simulink model "mrefrobotarm_previous_y_previous_u_previous_ref_cex_2"  (R2018b)
settings: Solver=FixedStepAuto  StartTime=0.0  StopTime=20  RelTol=1e-3  AbsTol=1e-6
undefined symbols (not defined in the file or in its folder): cc, options
libraries: neural x462, simulink x2
(part 14 of 18)

== system mrefrobotarm_previous_y_previous_u_previous_ref_cex_2/no_cex/Layer 3/Delays 1 ==
  "p{3}" : Inport  PortDimensions=30
      mask Display: e = 0.06;c1 = [120 230 180]/255;c2 = ([120 230 180]+0)/(256+128);c3 = ([120 230 180]+128)/(256+128);patch([0 1 1 0],[0 0 1 1],c1);patch([0 1 1 1-e 1-e 0+e],[0 0 1 1-e 0+e 0+e],c2);patch([0 0 1 1-e 0+e 0+e],[0 1 1 1-e 1-e 0+e],c3);plot([0 1 1 0 0],[0 0 1 1 0]);
  mux : Mux  Inputs=1
      mask Display: e = 0.06;c1 = [120 150 230]/255;c2 = ([120 150 230]+0)/383;c3 = ([120 150 230]+128)/383;patch([0 1 1 0],[0 0 1 1],c1);patch([0 1 1 1-e 1-e 0+e],[0 0 1 1-e 0+e 0+e],c2);patch([0 0 1 1-e 0+e 0+e],[0 1 1 1-e 1-e 0+e],c3);plot([0 1 1 0 0],[0 0 1 1 0]);disp('Mux')
  "pd{3,2}" : Outport
      mask Display: e = 0.06;c1 = [120 230 180]/255;c2 = ([120 230 180]+0)/(256+128);c3 = ([120 230 180]+128)/(256+128);patch([0 1 1 0],[0 0 1 1],c1);patch([0 1 1 1-e 1-e 0+e],[0 0 1 1-e 0+e 0+e],c2);patch([0 0 1 1-e 0+e 0+e],[0 1 1 1-e 1-e 0+e],c3);plot([0 1 1 0 0],[0 0 1 1 0]);
  wires:
  "p{3}"/1 -> mux/1
  mux/1 -> "pd{3,2}"/1

== system mrefrobotarm_previous_y_previous_u_previous_ref_cex_2/no_cex/Layer 3/LW{3,2} ==
  "ad{3,2}" : Inport  PortDimensions=30
      mask Display: e = 0.06;c1 = [120 230 180]/255;c2 = ([120 230 180]+0)/(256+128);c3 = ([120 230 180]+128)/(256+128);patch([0 1 1 0],[0 0 1 1],c1);patch([0 1 1 1-e 1-e 0+e],[0 0 1 1-e 0+e 0+e],c2);patch([0 0 1 1-e 0+e 0+e],[0 1 1 1-e 1-e 0+e],c3);plot([0 1 1 0 0],[0 0 1 1 0]);
  "IW{3,2}(1,:)'" : Constant  Value=[-0.179633159964680266806880126750911585986614227294921875;-0.01072873765062364037614628387018456123769283294677734375;-0.0291453057248748058360998669513719505630433559417724609375;0.05859045612955075810202032471352140419185161590576171875;-0.237638764700321913903025006220559589564800262451171875;-0.209838527725091539277713081901310943067073822021484375;-0.27791655307496510030063063823035918176174163818359375;-0.07008976059233355815347721318175899796187877655029296875;-0.11554327471293225626514100667918683029711246490478515625;0.27212249906517038677833397741778753697872161865234375;-0.1734031338030869451305449047140427865087985992431640625;0.0536763624525791460673218580268439836800098419189453125;-0.037173437880853761605681739865758572705090045928955078125;0.1358518131119930971717479906146763823926448822021484375;-0.11157815841815578450368917629020870663225650787353515625;-0.023913464068717076027592582931902143172919750213623046875;-0.4313994517536372530486232790281064808368682861328125;0.1636875861604869808463291747102630324661731719970703125;0.037232113811342650022684352961732656694948673248291015625;-0.52644415726454052428806562602403573691844940185546875;0.039897217969779720514456045066253864206373691558837890625;-0.1369287872106144388073545314910006709396839141845703125;0.44593864887069745162051503939437679946422576904296875;0.410742338437982856813590615274733863770961761474609375;-0.145121658875231818175421949490555562078952789306640625;0.06655502995710448066457587401600903831422328948974609375;-0.418109406113754300537976860141498036682605743408203125;0.11096998879556761730125202802810235880315303802490234375;0.333827163986122277261614499366260133683681488037109375;0.186101897373585012385177606120123527944087982177734375]
      mask Display: e = 0.06;c1 = [120 150 230]/255;c2 = ([120 150 230]+0)/383;c3 = ([120 150 230]+128)/383;patch([0 1 1 0],[0 0 1 1],c1);patch([0 1 1 1-e 1-e 0+e],[0 0 1 1-e 0+e 0+e],c2);patch([0 0 1 1-e 0+e 0+e],[0 1 1 1-e 1-e 0+e],c3);plot([0 1 1 0 0],[0 0 1 1 0]);disp('weights');
  Mux : Mux  Inputs=1
      mask Display: e = 0.06;c1 = [120 150 230]/255;c2 = ([120 150 230]+0)/383;c3 = ([120 150 230]+128)/383;patch([0 1 1 0],[0 0 1 1],c1);patch([0 1 1 1-e 1-e 0+e],[0 0 1 1-e 0+e 0+e],c2);patch([0 0 1 1-e 0+e 0+e],[0 1 1 1-e 1-e 0+e],c3);plot([0 1 1 0 0],[0 0 1 1 0]);disp('Mux');
  dotprod1 : neural/Weight Functions/dotprod
  "lz{3,2}" : Outport
      mask Display: e = 0.06;c1 = [120 230 180]/255;c2 = ([120 230 180]+0)/(256+128);c3 = ([120 230 180]+128)/(256+128);patch([0 1 1 0],[0 0 1 1],c1);patch([0 1 1 1-e 1-e 0+e],[0 0 1 1-e 0+e 0+e],c2);patch([0 0 1 1-e 0+e 0+e],[0 1 1 1-e 1-e 0+e],c3);plot([0 1 1 0 0],[0 0 1 1 0]);
  wires:
  "IW{3,2}(1,:)'"/1 -> dotprod1/1
  "ad{3,2}"/1 -> dotprod1/2
  dotprod1/1 -> Mux/1
  Mux/1 -> "lz{3,2}"/1

== system mrefrobotarm_previous_y_previous_u_previous_ref_cex_2/no_cex1/Layer 1/Delays 1 ==
  "p{1}" : Inport  PortDimensions=10
      mask Display: e = 0.06;c1 = [120 230 180]/255;c2 = ([120 230 180]+0)/(256+128);c3 = ([120 230 180]+128)/(256+128);patch([0 1 1 0],[0 0 1 1],c1);patch([0 1 1 1-e 1-e 0+e],[0 0 1 1-e 0+e 0+e],c2);patch([0 0 1 1-e 0+e 0+e],[0 1 1 1-e 1-e 0+e],c3);plot([0 1 1 0 0],[0 0 1 1 0]);
  mux : Mux  Inputs=1
      mask Display: e = 0.06;c1 = [120 150 230]/255;c2 = ([120 150 230]+0)/383;c3 = ([120 150 230]+128)/383;patch([0 1 1 0],[0 0 1 1],c1);patch([0 1 1 1-e 1-e 0+e],[0 0 1 1-e 0+e 0+e],c2);patch([0 0 1 1-e 0+e 0+e],[0 1 1 1-e 1-e 0+e],c3);plot([0 1 1 0 0],[0 0 1 1 0]);disp('Mux')
  "pd{1,1}" : Outport
      mask Display: e = 0.06;c1 = [120 230 180]/255;c2 = ([120 230 180]+0)/(256+128);c3 = ([120 230 180]+128)/(256+128);patch([0 1 1 0],[0 0 1 1],c1);patch([0 1 1 1-e 1-e 0+e],[0 0 1 1-e 0+e 0+e],c2);patch([0 0 1 1-e 0+e 0+e],[0 1 1 1-e 1-e 0+e],c3);plot([0 1 1 0 0],[0 0 1 1 0]);
  wires:
  "p{1}"/1 -> mux/1
  mux/1 -> "pd{1,1}"/1

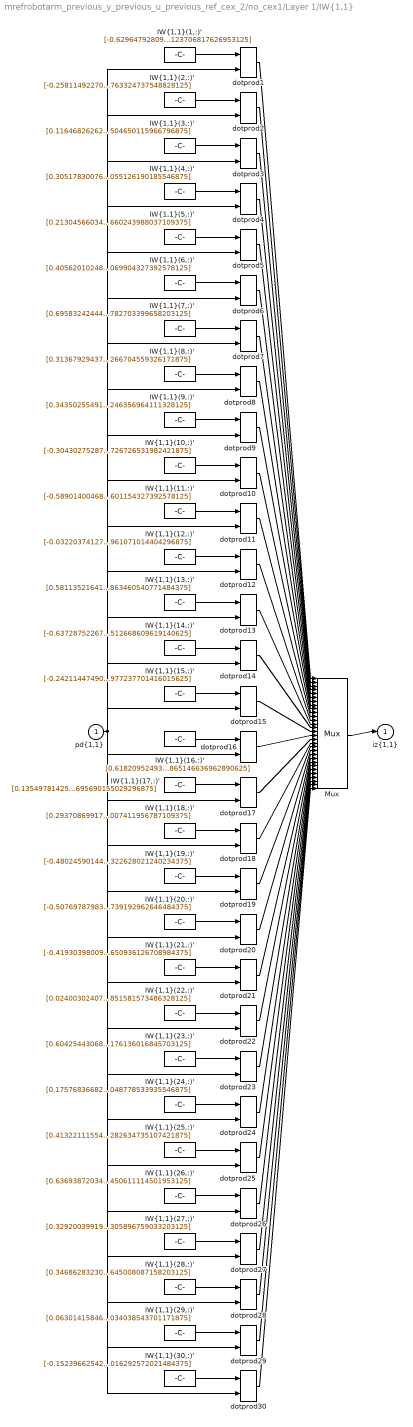
== system mrefrobotarm_previous_y_previous_u_previous_ref_cex_2/no_cex1/Layer 1/IW{1,1} ==
  "pd{1,1}" : Inport  PortDimensions=10
      mask Display: e = 0.06;c1 = [120 230 180]/255;c2 = ([120 230 180]+0)/(256+128);c3 = ([120 230 180]+128)/(256+128);patch([0 1 1 0],[0 0 1 1],c1);patch([0 1 1 1-e 1-e 0+e],[0 0 1 1-e 0+e 0+e],c2);patch([0 0 1 1-e 0+e 0+e],[0 1 1 1-e 1-e 0+e],c3);plot([0 1 1 0 0],[0 0 1 1 0]);
  "IW{1,1}(1,:)'" : Constant  Value=[-0.6296479280930478150679618920548819005489349365234375;0.01798174319361729722732690106568043120205402374267578125;0.749989571787455844287251238711178302764892578125;-0.126212854667532681229857871585409156978130340576171875;0.09955965014467361984262794294409104622900485992431640625;-0.497213497116828662125698201634804718196392059326171875;0.245933783155573404410887405902030877768993377685546875;-0.14626152846809958862905887144734151661396026611328125;0.191256073096406797873214600258506834506988525390625;-0.541272076643626309788714934256859123706817626953125]
      mask Display: e = 0.06;c1 = [120 150 230]/255;c2 = ([120 150 230]+0)/383;c3 = ([120 150 230]+128)/383;patch([0 1 1 0],[0 0 1 1],c1);patch([0 1 1 1-e 1-e 0+e],[0 0 1 1-e 0+e 0+e],c2);patch([0 0 1 1-e 0+e 0+e],[0 1 1 1-e 1-e 0+e],c3);plot([0 1 1 0 0],[0 0 1 1 0]);disp('Weights');
  "IW{1,1}(10,:)'" : Constant  Value=[-0.304302752876717430563502375662210397422313690185546875;0.19061480666327590416386783545021899044513702392578125;-0.0186846885284801221549511041075675166212022304534912109375;-0.0797161528025709109623875292527372948825359344482421875;0.467056189107703467744414638218586333096027374267578125;0.3914649652758408482355889645987190306186676025390625;-0.411903997528578036391166961038834415376186370849609375;0.36287834914432881561197064002044498920440673828125;-0.67254358864622887370643411486526019871234893798828125;-0.46317281151571243480447037654812447726726531982421875]
      mask Display: e = 0.06;c1 = [120 150 230]/255;c2 = ([120 150 230]+0)/383;c3 = ([120 150 230]+128)/383;patch([0 1 1 0],[0 0 1 1],c1);patch([0 1 1 1-e 1-e 0+e],[0 0 1 1-e 0+e 0+e],c2);patch([0 0 1 1-e 0+e 0+e],[0 1 1 1-e 1-e 0+e],c3);plot([0 1 1 0 0],[0 0 1 1 0]);disp('Weights');
  "IW{1,1}(11,:)'" : Constant  Value=[-0.589014004683919178972928420989774167537689208984375;0.424032911647191534942891166792833246290683746337890625;-0.437906224214046291276503097833483479917049407958984375;0.5688051621976260019408755397307686507701873779296875;-0.38519457534442824719889131301897577941417694091796875;-0.54092808591898633441275023869820870459079742431640625;0.1918827885460951676588337022621999494731426239013671875;0.2418540370781511461562018894255743362009525299072265625;0.287848556840362868047833444506977684795856475830078125;0.26019956067512595154767041094601154327392578125]
      mask Display: e = 0.06;c1 = [120 150 230]/255;c2 = ([120 150 230]+0)/383;c3 = ([120 150 230]+128)/383;patch([0 1 1 0],[0 0 1 1],c1);patch([0 1 1 1-e 1-e 0+e],[0 0 1 1-e 0+e 0+e],c2);patch([0 0 1 1-e 0+e 0+e],[0 1 1 1-e 1-e 0+e],c3);plot([0 1 1 0 0],[0 0 1 1 0]);disp('Weights');
  "IW{1,1}(12,:)'" : Constant  Value=[-0.032203741273671683542634269770132959820330142974853515625;0.46435771114908253043296326723066158592700958251953125;-0.40490000280688065448231327536632306873798370361328125;0.58373729678087393768493029710953123867511749267578125;0.5665227535105070710841346226516179740428924560546875;-0.74861259763472831618713598800241015851497650146484375;0.06260189988691709783719119286615750752389430999755859375;-0.3281222927468883110435626804246567189693450927734375;0.10700863518534968477080582260896335355937480926513671875;0.196892455182014092240905256403493694961071014404296875]
      mask Display: e = 0.06;c1 = [120 150 230]/255;c2 = ([120 150 230]+0)/383;c3 = ([120 150 230]+128)/383;patch([0 1 1 0],[0 0 1 1],c1);patch([0 1 1 1-e 1-e 0+e],[0 0 1 1-e 0+e 0+e],c2);patch([0 0 1 1-e 0+e 0+e],[0 1 1 1-e 1-e 0+e],c3);plot([0 1 1 0 0],[0 0 1 1 0]);disp('Weights');
  "IW{1,1}(13,:)'" : Constant  Value=[0.58113521641844567700019297262770123779773712158203125;-0.6340777353433566521090369860758073627948760986328125;0.2343980124863034031346131769169005565345287322998046875;0.5373827789826182144139465890475548803806304931640625;-0.2056939980958405189692683734392630867660045623779296875;0.54163935118717920769171314532286487519741058349609375;-0.465711998386639736136061173965572379529476165771484375;-0.400154676589407787279384365319856442511081695556640625;-0.1149558097368235942692393791730864904820919036865234375;-0.038427729017857702176197420840253471396863460540771484375]
      mask Display: e = 0.06;c1 = [120 150 230]/255;c2 = ([120 150 230]+0)/383;c3 = ([120 150 230]+128)/383;patch([0 1 1 0],[0 0 1 1],c1);patch([0 1 1 1-e 1-e 0+e],[0 0 1 1-e 0+e 0+e],c2);patch([0 0 1 1-e 0+e 0+e],[0 1 1 1-e 1-e 0+e],c3);plot([0 1 1 0 0],[0 0 1 1 0]);disp('Weights');
  "IW{1,1}(14,:)'" : Constant  Value=[-0.63728752267550314858368665227317251265048980712890625;-0.30135663453486782881185490623465739190578460693359375;0.052250715025683826253644070902737439610064029693603515625;-0.1726020371843388356847270870275679044425487518310546875;0.365826182343079120418138927561813034117221832275390625;0.55077737774850987761965370737016201019287109375;0.28906499312449496219556976939202286303043365478515625;-0.5791735820286436631221249626833014190196990966796875;0.60966753205327972597871166726690717041492462158203125;0.387731198834659895879894975223578512668609619140625]
      mask Display: e = 0.06;c1 = [120 150 230]/255;c2 = ([120 150 230]+0)/383;c3 = ([120 150 230]+128)/383;patch([0 1 1 0],[0 0 1 1],c1);patch([0 1 1 1-e 1-e 0+e],[0 0 1 1-e 0+e 0+e],c2);patch([0 0 1 1-e 0+e 0+e],[0 1 1 1-e 1-e 0+e],c3);plot([0 1 1 0 0],[0 0 1 1 0]);disp('Weights');
  "IW{1,1}(15,:)'" : Constant  Value=[-0.2421144749092230818998672248199000023305416107177734375;-0.11567718586728918672701382774903322570025920867919921875;0.38155440532766682348864151208545081317424774169921875;0.023609431528087455876008249333608546294271945953369140625;-0.540832332461979259363715755171142518520355224609375;-0.222867819913187215075112135309609584510326385498046875;-0.08659947127838972524838112576617277227342128753662109375;-0.675898932576143085526609866064973175525665283203125;-0.797880071334330143173474425566382706165313720703125;-0.28873160017808940924766147873015142977237701416015625]
      mask Display: e = 0.06;c1 = [120 150 230]/255;c2 = ([120 150 230]+0)/383;c3 = ([120 150 230]+128)/383;patch([0 1 1 0],[0 0 1 1],c1);patch([0 1 1 1-e 1-e 0+e],[0 0 1 1-e 0+e 0+e],c2);patch([0 0 1 1-e 0+e 0+e],[0 1 1 1-e 1-e 0+e],c3);plot([0 1 1 0 0],[0 0 1 1 0]);disp('Weights');
  "IW{1,1}(16,:)'" : Constant  Value=[0.61820952493411029937675493783899582922458648681640625;-0.50802521912933229497610909675131551921367645263671875;0.57134809831430810600494396567228250205516815185546875;0.5712105054721827723795968267950229346752166748046875;-0.38637038016985181254625558722182177007198333740234375;0.139540503933613557752124734179233200848102569580078125;0.4215957486368118178887698377366177737712860107421875;-0.1279673121080379394332027231939719058573246002197265625;-0.1311627739086217159236724683069041930139064788818359375;0.16557349416556699228664228940033353865146636962890625]
      mask Display: e = 0.06;c1 = [120 150 230]/255;c2 = ([120 150 230]+0)/383;c3 = ([120 150 230]+128)/383;patch([0 1 1 0],[0 0 1 1],c1);patch([0 1 1 1-e 1-e 0+e],[0 0 1 1-e 0+e 0+e],c2);patch([0 0 1 1-e 0+e 0+e],[0 1 1 1-e 1-e 0+e],c3);plot([0 1 1 0 0],[0 0 1 1 0]);disp('Weights');
  "IW{1,1}(17,:)'" : Constant  Value=[0.13549781425094753473103992291726171970367431640625;-0.5072485017807775165010752971284091472625732421875;0.436861760574706770032804570291773416101932525634765625;-0.43770890890160496500271847253316082060337066650390625;-0.45041635586474992880567924657952971756458282470703125;-0.430649769874818011405892548282281495630741119384765625;0.002995504803380683554736574336629928438924252986907958984375;-0.59460351282356327384803762470255605876445770263671875;-0.55740200379700077792932688680593855679035186767578125;-0.007037453928122709700954118261506664566695690155029296875]
      mask Display: e = 0.06;c1 = [120 150 230]/255;c2 = ([120 150 230]+0)/383;c3 = ([120 150 230]+128)/383;patch([0 1 1 0],[0 0 1 1],c1);patch([0 1 1 1-e 1-e 0+e],[0 0 1 1-e 0+e 0+e],c2);patch([0 0 1 1-e 0+e 0+e],[0 1 1 1-e 1-e 0+e],c3);plot([0 1 1 0 0],[0 0 1 1 0]);disp('Weights');
  "IW{1,1}(18,:)'" : Constant  Value=[0.293708699173908349688844054981018416583538055419921875;-0.31855962054320918763750114521826617419719696044921875;0.3123496018616280789359507252811454236507415771484375;0.0127261086725141935038774221311541623435914516448974609375;-0.392332467634265824596440097593585960566997528076171875;0.3062597653282936871477204476832412183284759521484375;-0.28089761551940028994067688472568988800048828125;0.071330191199411585589729156708926893770694732666015625;0.7530176231304424039336709029157646000385284423828125;0.95183623378654080848804142078734003007411956787109375]
      mask Display: e = 0.06;c1 = [120 150 230]/255;c2 = ([120 150 230]+0)/383;c3 = ([120 150 230]+128)/383;patch([0 1 1 0],[0 0 1 1],c1);patch([0 1 1 1-e 1-e 0+e],[0 0 1 1-e 0+e 0+e],c2);patch([0 0 1 1-e 0+e 0+e],[0 1 1 1-e 1-e 0+e],c3);plot([0 1 1 0 0],[0 0 1 1 0]);disp('Weights');
  "IW{1,1}(19,:)'" : Constant  Value=[-0.480245901444267653257469419258995912969112396240234375;-0.53326159497092906480730789553490467369556427001953125;-0.323673669420163900856124428173643536865711212158203125;-0.2427693724438767242101988586000516079366207122802734375;-0.1277519244074492299478862378236954100430011749267578125;-0.07393542742682733537318284788852906785905361175537109375;0.27023740710218124849717469260212965309619903564453125;-0.48991768470402730084600761983892880380153656005859375;-0.476314019055344706199406346058822236955165863037109375;0.2396832333781181156862061243373318575322628021240234375]
      mask Display: e = 0.06;c1 = [120 150 230]/255;c2 = ([120 150 230]+0)/383;c3 = ([120 150 230]+128)/383;patch([0 1 1 0],[0 0 1 1],c1);patch([0 1 1 1-e 1-e 0+e],[0 0 1 1-e 0+e 0+e],c2);patch([0 0 1 1-e 0+e 0+e],[0 1 1 1-e 1-e 0+e],c3);plot([0 1 1 0 0],[0 0 1 1 0]);disp('Weights');
  "IW{1,1}(2,:)'" : Constant  Value=[-0.25811492270229308143569824096630327403545379638671875;-0.2471154463373592680142110111773945391178131103515625;0.25818043542167534720732646746910177171230316162109375;0.375392581149148363284240303983096964657306671142578125;-0.1667489954308243038649806067041936330497264862060546875;-0.4474564798920044328411904643871821463108062744140625;-0.49749250577287995600528347495128400623798370361328125;0.526766359274847051352708149352110922336578369140625;0.49941063626364223804188213762245140969753265380859375;0.426177216245306411668281043603201396763324737548828125]
      mask Display: e = 0.06;c1 = [120 150 230]/255;c2 = ([120 150 230]+0)/383;c3 = ([120 150 230]+128)/383;patch([0 1 1 0],[0 0 1 1],c1);patch([0 1 1 1-e 1-e 0+e],[0 0 1 1-e 0+e 0+e],c2);patch([0 0 1 1-e 0+e 0+e],[0 1 1 1-e 1-e 0+e],c3);plot([0 1 1 0 0],[0 0 1 1 0]);disp('Weights');
  "IW{1,1}(20,:)'" : Constant  Value=[-0.507697879834486887062894311384297907352447509765625;-0.323457740498831192166306891522253863513469696044921875;-0.53597473743813583979545001056976616382598876953125;0.342750671651670668627076565826428122818470001220703125;0.382564898254284024847748924003099091351032257080078125;0.034243898078243774352191763910013833083212375640869140625;0.277233785624469597497210315850679762661457061767578125;-0.366259036140992033647734160695108585059642791748046875;-0.462643611474350124890264623900293372571468353271484375;-0.3712129121769167650057852370082400739192962646484375]
      mask Display: e = 0.06;c1 = [120 150 230]/255;c2 = ([120 150 230]+0)/383;c3 = ([120 150 230]+128)/383;patch([0 1 1 0],[0 0 1 1],c1);patch([0 1 1 1-e 1-e 0+e],[0 0 1 1-e 0+e 0+e],c2);patch([0 0 1 1-e 0+e 0+e],[0 1 1 1-e 1-e 0+e],c3);plot([0 1 1 0 0],[0 0 1 1 0]);disp('Weights');
  "IW{1,1}(21,:)'" : Constant  Value=[-0.419303980098666928544304255410679616034030914306640625;0.0685480105728574484746928874301374889910221099853515625;0.450858230972308871020715059785288758575916290283203125;0.43708869281008466689542046879068948328495025634765625;-0.29432151962089381225240458661573939025402069091796875;0.458506040966411954062920131036662496626377105712890625;-0.29492393095573554706589902707492001354694366455078125;0.0906994943155156885250534060105565004050731658935546875;-0.227334062327028962879893470017123036086559295654296875;0.6843549578157082091678375945775769650936126708984375]
      mask Display: e = 0.06;c1 = [120 150 230]/255;c2 = ([120 150 230]+0)/383;c3 = ([120 150 230]+128)/383;patch([0 1 1 0],[0 0 1 1],c1);patch([0 1 1 1-e 1-e 0+e],[0 0 1 1-e 0+e 0+e],c2);patch([0 0 1 1-e 0+e 0+e],[0 1 1 1-e 1-e 0+e],c3);plot([0 1 1 0 0],[0 0 1 1 0]);disp('Weights');
  "IW{1,1}(22,:)'" : Constant  Value=[0.0240030240768657303351840681671092170290648937225341796875;0.1781395962941281496672019102334161289036273956298828125;0.639385027599914668172687015612609684467315673828125;0.577242713304108701066752473707310855388641357421875;0.33420283979382536809765724683529697358608245849609375;0.002297073726901973679537238837156110093928873538970947265625;-0.05484687515281870540118092094417079351842403411865234375;-0.13085772587827981805475019427831284701824188232421875;0.546714955350407816325741805485449731349945068359375;0.55485118173807734809344083259929902851581573486328125]
      mask Display: e = 0.06;c1 = [120 150 230]/255;c2 = ([120 150 230]+0)/383;c3 = ([120 150 230]+128)/383;patch([0 1 1 0],[0 0 1 1],c1);patch([0 1 1 1-e 1-e 0+e],[0 0 1 1-e 0+e 0+e],c2);patch([0 0 1 1-e 0+e 0+e],[0 1 1 1-e 1-e 0+e],c3);plot([0 1 1 0 0],[0 0 1 1 0]);disp('Weights');
  "IW{1,1}(23,:)'" : Constant  Value=[0.60425443068960638104414329063729383051395416259765625;0.53667490374154735999212562091997824609279632568359375;0.29268345212147017786463720767642371356487274169921875;0.319047492023566470198403521862928755581378936767578125;0.191898791278704072826855053790495730936527252197265625;0.045254192335671787617012995497134397737681865692138671875;0.4280331193524957722473800458828918635845184326171875;0.58314504141383360913408751002862118184566497802734375;-0.31818874162630184088129681185819208621978759765625;0.5414335954602276235192448439192958176136016845703125]
      mask Display: e = 0.06;c1 = [120 150 230]/255;c2 = ([120 150 230]+0)/383;c3 = ([120 150 230]+128)/383;patch([0 1 1 0],[0 0 1 1],c1);patch([0 1 1 1-e 1-e 0+e],[0 0 1 1-e 0+e 0+e],c2);patch([0 0 1 1-e 0+e 0+e],[0 1 1 1-e 1-e 0+e],c3);plot([0 1 1 0 0],[0 0 1 1 0]);disp('Weights');
  "IW{1,1}(24,:)'" : Constant  Value=[0.1757683668273537780368798166819033212959766387939453125;0.28174477295346023186795036963303573429584503173828125;-0.0669749020800512184781183577797492034733295440673828125;-0.0930431689804126771381476146416389383375644683837890625;0.50026413726126783831915645350818522274494171142578125;-0.6475724813899057519250845871283672749996185302734375;0.1709767738480999221817313582505448721349239349365234375;-0.5982369798411231176515912011382170021533966064453125;0.160595631110304892796847298086504451930522918701171875;0.4941363635631415007765099289827048778533935546875]
      mask Display: e = 0.06;c1 = [120 150 230]/255;c2 = ([120 150 230]+0)/383;c3 = ([120 150 230]+128)/383;patch([0 1 1 0],[0 0 1 1],c1);patch([0 1 1 1-e 1-e 0+e],[0 0 1 1-e 0+e 0+e],c2);patch([0 0 1 1-e 0+e 0+e],[0 1 1 1-e 1-e 0+e],c3);plot([0 1 1 0 0],[0 0 1 1 0]);disp('Weights');
  "IW{1,1}(25,:)'" : Constant  Value=[0.4132211155410880909499837798648513853549957275390625;0.464236894342753225739528488702489994466304779052734375;-0.15895974992269634729069593959138728678226470947265625;-0.59574810817631795867299615565571002662181854248046875;-0.042943129182051516246065858695146744139492511749267578125;-0.397791091329356694128449589697993360459804534912109375;-0.490360603100838676748907118962961249053478240966796875;-0.45577915993366036051526180017390288412570953369140625;-0.1067305977679246786760103304914082400500774383544921875;0.306373288959848444346079077149624936282634735107421875]
      mask Display: e = 0.06;c1 = [120 150 230]/255;c2 = ([120 150 230]+0)/383;c3 = ([120 150 230]+128)/383;patch([0 1 1 0],[0 0 1 1],c1);patch([0 1 1 1-e 1-e 0+e],[0 0 1 1-e 0+e 0+e],c2);patch([0 0 1 1-e 0+e 0+e],[0 1 1 1-e 1-e 0+e],c3);plot([0 1 1 0 0],[0 0 1 1 0]);disp('Weights');
  "IW{1,1}(26,:)'" : Constant  Value=[0.6369387203462004709564325821702368557453155517578125;0.79380248937343289572510229845647700130939483642578125;0.00164302389077067832225120813660623753094114363193511962890625;-0.27336353690975767616322400499484501779079437255859375;-0.26618290065019201140472659972147084772586822509765625;0.0320094835373095631947393258087686263024806976318359375;-0.423526012306385146732878865805105306208133697509765625;-0.326830052302183371448762727595749311149120330810546875;0.1613767113064828173651932274879072792828083038330078125;0.0982428865021336694685061274867621250450611114501953125]
      mask Display: e = 0.06;c1 = [120 150 230]/255;c2 = ([120 150 230]+0)/383;c3 = ([120 150 230]+128)/383;patch([0 1 1 0],[0 0 1 1],c1);patch([0 1 1 1-e 1-e 0+e],[0 0 1 1-e 0+e 0+e],c2);patch([0 0 1 1-e 0+e 0+e],[0 1 1 1-e 1-e 0+e],c3);plot([0 1 1 0 0],[0 0 1 1 0]);disp('Weights');
  "IW{1,1}(27,:)'" : Constant  Value=[0.329200399195510085004201528136036358773708343505859375;0.28287689109151992195023694875999353826045989990234375;-0.4847213207485039365707280012429691851139068603515625;-0.1284411255237942472984258301949012093245983123779296875;-0.174015706102306044744665314283338375389575958251953125;-0.329651737080481066488601982200634665787220001220703125;-0.168014111647432795582091102915001101791858673095703125;-0.334496503872005579438564382144249975681304931640625;-0.58085869426907510426616454424220137298107147216796875;0.69699734974279448085354715658468194305896759033203125]
      mask Display: e = 0.06;c1 = [120 150 230]/255;c2 = ([120 150 230]+0)/383;c3 = ([120 150 230]+128)/383;patch([0 1 1 0],[0 0 1 1],c1);patch([0 1 1 1-e 1-e 0+e],[0 0 1 1-e 0+e 0+e],c2);patch([0 0 1 1-e 0+e 0+e],[0 1 1 1-e 1-e 0+e],c3);plot([0 1 1 0 0],[0 0 1 1 0]);disp('Weights');
  "IW{1,1}(28,:)'" : Constant  Value=[0.3468628323059610440992628355161286890506744384765625;0.0268740280843508365371530288712165202014148235321044921875;0.25601058258245334986469288196531124413013458251953125;-0.3437401579640899651479912790819071233272552490234375;0.4867288533715965481718512819497846066951751708984375;-0.184162904833906682089406103841611184179782867431640625;0.67145036486717735169094112279708497226238250732421875;-0.372284944733178135845008682736079208552837371826171875;-0.1119306956150517839976288314574048854410648345947265625;0.2384872923248953224817370255550486035645008087158203125]
      mask Display: e = 0.06;c1 = [120 150 230]/255;c2 = ([120 150 230]+0)/383;c3 = ([120 150 230]+128)/383;patch([0 1 1 0],[0 0 1 1],c1);patch([0 1 1 1-e 1-e 0+e],[0 0 1 1-e 0+e 0+e],c2);patch([0 0 1 1-e 0+e 0+e],[0 1 1 1-e 1-e 0+e],c3);plot([0 1 1 0 0],[0 0 1 1 0]);disp('Weights');
  "IW{1,1}(29,:)'" : Constant  Value=[0.06301415846665082975963656508611165918409824371337890625;-0.10825577920747797566747294695232994854450225830078125;-0.5771167653503186389940537992515601217746734619140625;-0.387661968548416002722234452448901720345020294189453125;-0.125723671682269222404926267699920572340488433837890625;-0.60714349894266483875782114409958012402057647705078125;-0.043044947809864557430881149002743768505752086639404296875;0.378712978917156439795377309565083123743534088134765625;-0.643524128456367083828126851585693657398223876953125;-0.419458376014482936522398404122213833034038543701171875]
      mask Display: e = 0.06;c1 = [120 150 230]/255;c2 = ([120 150 230]+0)/383;c3 = ([120 150 230]+128)/383;patch([0 1 1 0],[0 0 1 1],c1);patch([0 1 1 1-e 1-e 0+e],[0 0 1 1-e 0+e 0+e],c2);patch([0 0 1 1-e 0+e 0+e],[0 1 1 1-e 1-e 0+e],c3);plot([0 1 1 0 0],[0 0 1 1 0]);disp('Weights');
  "IW{1,1}(3,:)'" : Constant  Value=[0.1164682626283675970224606999181560240685939788818359375;0.283807095653487884145960151727194897830486297607421875;-0.274985771002521584005506838366272859275341033935546875;0.0650003452624407784821158884369651786983013153076171875;0.292159300924412168587451787971076555550098419189453125;-0.450263090761314599408393632984370924532413482666015625;0.364462506083464476969169254516600631177425384521484375;-0.1974066741664597113281587326127919368445873260498046875;0.58064414825165344691271229748963378369808197021484375;-0.65405849178335262461558841096120886504650115966796875]
      mask Display: e = 0.06;c1 = [120 150 230]/255;c2 = ([120 150 230]+0)/383;c3 = ([120 150 230]+128)/383;patch([0 1 1 0],[0 0 1 1],c1);patch([0 1 1 1-e 1-e 0+e],[0 0 1 1-e 0+e 0+e],c2);patch([0 0 1 1-e 0+e 0+e],[0 1 1 1-e 1-e 0+e],c3);plot([0 1 1 0 0],[0 0 1 1 0]);disp('Weights');
  "IW{1,1}(30,:)'" : Constant  Value=[-0.1523966254235673556394203842501156032085418701171875;-0.50914859959029945546404860579059459269046783447265625;-0.62916922137648523261077571078203618526458740234375;0.5050572709087755018941834350698627531528472900390625;-0.39851089475858059163471125430078245699405670166015625;0.3379244782851202888451780381728895008563995361328125;0.2011112653232325631069699056752142496407032012939453125;-0.245693538789234278141293543740175664424896240234375;0.050319182148697259859826402816906920634210109710693359375;0.28919329169113738853269524042843841016292572021484375]
      mask Display: e = 0.06;c1 = [120 150 230]/255;c2 = ([120 150 230]+0)/383;c3 = ([120 150 230]+128)/383;patch([0 1 1 0],[0 0 1 1],c1);patch([0 1 1 1-e 1-e 0+e],[0 0 1 1-e 0+e 0+e],c2);patch([0 0 1 1-e 0+e 0+e],[0 1 1 1-e 1-e 0+e],c3);plot([0 1 1 0 0],[0 0 1 1 0]);disp('Weights');
  "IW{1,1}(4,:)'" : Constant  Value=[0.305178300764842147518862702781916595995426177978515625;-0.480747829516201263810870614179293625056743621826171875;0.70946132259131544639529920459608547389507293701171875;0.00658407173914657938007533033442086889408528804779052734375;0.282976336902390601668599856566288508474826812744140625;-0.333564766752495522883492640175973065197467803955078125;0.2496429672599569105084782449921476654708385467529296875;0.1985801323522411454547409448423422873020172119140625;0.0959957759015966083371296235782210715115070343017578125;0.554396002235488349896286308648996055126190185546875]
      mask Display: e = 0.06;c1 = [120 150 230]/255;c2 = ([120 150 230]+0)/383;c3 = ([120 150 230]+128)/383;patch([0 1 1 0],[0 0 1 1],c1);patch([0 1 1 1-e 1-e 0+e],[0 0 1 1-e 0+e 0+e],c2);patch([0 0 1 1-e 0+e 0+e],[0 1 1 1-e 1-e 0+e],c3);plot([0 1 1 0 0],[0 0 1 1 0]);disp('Weights');
  "IW{1,1}(5,:)'" : Constant  Value=[0.2130456603428758366458595219228300265967845916748046875;-0.626212866692530401024896491435356438159942626953125;0.62307138820618634955650350093492306768894195556640625;-0.15596731886291814728195959105505608022212982177734375;0.46757865976194123991405149354250170290470123291015625;0.54445080818472801897911494961590506136417388916015625;-0.1897793500678525979719069027851219289004802703857421875;-0.267266873315657405019152292879880405962467193603515625;0.2212324237810018578986870352309779264032840728759765625;0.0627108044427452104851994363343692384660243988037109375]
      mask Display: e = 0.06;c1 = [120 150 230]/255;c2 = ([120 150 230]+0)/383;c3 = ([120 150 230]+128)/383;patch([0 1 1 0],[0 0 1 1],c1);patch([0 1 1 1-e 1-e 0+e],[0 0 1 1-e 0+e 0+e],c2);patch([0 0 1 1-e 0+e 0+e],[0 1 1 1-e 1-e 0+e],c3);plot([0 1 1 0 0],[0 0 1 1 0]);disp('Weights');
  "IW{1,1}(6,:)'" : Constant  Value=[0.405620102489697043068872517324052751064300537109375;-0.1530449384935525791728849753781105391681194305419921875;-0.2029659900349511103545552259674877859652042388916015625;-0.052779101938537319183009088874314329586923122406005859375;-0.25094393784506785483046087392722256481647491455078125;0.61749021472933918186498658542404882609844207763671875;-0.10381910600384815224206391803818405605852603912353515625;-0.5146000583413741225058402051217854022979736328125;-0.490082572628723678320739054470323026180267333984375;-0.1841894416331388839580540661700069904327392578125]
      mask Display: e = 0.06;c1 = [120 150 230]/255;c2 = ([120 150 230]+0)/383;c3 = ([120 150 230]+128)/383;patch([0 1 1 0],[0 0 1 1],c1);patch([0 1 1 1-e 1-e 0+e],[0 0 1 1-e 0+e 0+e],c2);patch([0 0 1 1-e 0+e 0+e],[0 1 1 1-e 1-e 0+e],c3);plot([0 1 1 0 0],[0 0 1 1 0]);disp('Weights');
  "IW{1,1}(7,:)'" : Constant  Value=[0.69583242444276793836621664013364352285861968994140625;0.301376531380843803997748864276218228042125701904296875;-0.445025429800517680067883929950767196714878082275390625;-0.53749242302939126414429438227671198546886444091796875;-0.2345704502368468336026552378825726918876171112060546875;-0.02426772144156974508888424679753370583057403564453125;-0.07265836875424837304482394984006532467901706695556640625;-0.1819706025522481451783818329204223118722438812255859375;0.411732245476257474603443142768810503184795379638671875;0.374529852191533063621164956202846951782703399658203125]
      mask Display: e = 0.06;c1 = [120 150 230]/255;c2 = ([120 150 230]+0)/383;c3 = ([120 150 230]+128)/383;patch([0 1 1 0],[0 0 1 1],c1);patch([0 1 1 1-e 1-e 0+e],[0 0 1 1-e 0+e 0+e],c2);patch([0 0 1 1-e 0+e 0+e],[0 1 1 1-e 1-e 0+e],c3);plot([0 1 1 0 0],[0 0 1 1 0]);disp('Weights');
  "IW{1,1}(8,:)'" : Constant  Value=[0.3136792943753992091160398558713495731353759765625;-0.38702258946604983780304110041470266878604888916015625;-0.050657303550427190685923051205463707447052001953125;0.1313159503915729275913548690368770621716976165771484375;0.272553068767638517755358407157473266124725341796875;-0.10766861625745656472208366949416813440620899200439453125;-0.6098668815054371084016793247428722679615020751953125;0.53915474544308394921898752727429382503032684326171875;-0.5041014672225296866514554494642652571201324462890625;0.58201797497755947130571030356804840266704559326171875]
      mask Display: e = 0.06;c1 = [120 150 230]/255;c2 = ([120 150 230]+0)/383;c3 = ([120 150 230]+128)/383;patch([0 1 1 0],[0 0 1 1],c1);patch([0 1 1 1-e 1-e 0+e],[0 0 1 1-e 0+e 0+e],c2);patch([0 0 1 1-e 0+e 0+e],[0 1 1 1-e 1-e 0+e],c3);plot([0 1 1 0 0],[0 0 1 1 0]);disp('Weights');
  "IW{1,1}(9,:)'" : Constant  Value=[0.343502554919040303804678160304320044815540313720703125;-0.2782376252001206307085112712229602038860321044921875;-0.699781310856858684843473383807577192783355712890625;0.208434736990827484959254434215836226940155029296875;-0.0415256568078336829596963752919691614806652069091796875;-0.30957905234634586211228679530904628336429595947265625;-0.57936051835488766581505615249625407159328460693359375;-0.44983986077959825511385361096472479403018951416015625;-0.555030381678020656721628256491385400295257568359375;0.129335515216769891821968485601246356964111328125]
      mask Display: e = 0.06;c1 = [120 150 230]/255;c2 = ([120 150 230]+0)/383;c3 = ([120 150 230]+128)/383;patch([0 1 1 0],[0 0 1 1],c1);patch([0 1 1 1-e 1-e 0+e],[0 0 1 1-e 0+e 0+e],c2);patch([0 0 1 1-e 0+e 0+e],[0 1 1 1-e 1-e 0+e],c3);plot([0 1 1 0 0],[0 0 1 1 0]);disp('Weights');
  Mux : Mux  Inputs=30
      mask Display: e = 0.06;c1 = [120 150 230]/255;c2 = ([120 150 230]+0)/383;c3 = ([120 150 230]+128)/383;patch([0 1 1 0],[0 0 1 1],c1);patch([0 1 1 1-e 1-e 0+e],[0 0 1 1-e 0+e 0+e],c2);patch([0 0 1 1-e 0+e 0+e],[0 1 1 1-e 1-e 0+e],c3);plot([0 1 1 0 0],[0 0 1 1 0]);disp('Mux');
  dotprod{1..30} (30 alike) : neural/Weight Functions/dotprod
  "iz{1,1}" : Outport
      mask Display: e = 0.06;c1 = [120 230 180]/255;c2 = ([120 230 180]+0)/(256+128);c3 = ([120 230 180]+128)/(256+128);patch([0 1 1 0],[0 0 1 1],c1);patch([0 1 1 1-e 1-e 0+e],[0 0 1 1-e 0+e 0+e],c2);patch([0 0 1 1-e 0+e 0+e],[0 1 1 1-e 1-e 0+e],c3);plot([0 1 1 0 0],[0 0 1 1 0]);
  wires:
  "IW{1,1}(1,:)'"/1 -> dotprod1/1
  "pd{1,1}"/1 -> dotprod1/2, dotprod2/2, dotprod3/2, dotprod4/2, dotprod5/2, dotprod6/2, dotprod7/2, dotprod8/2, dotprod9/2, dotprod10/2, dotprod11/2, dotprod12/2, dotprod13/2, dotprod14/2, dotprod15/2, dotprod16/2, dotprod17/2, dotprod18/2, dotprod19/2, dotprod20/2, dotprod21/2, dotprod22/2, dotprod23/2, dotprod24/2, dotprod25/2, dotprod26/2, dotprod27/2, dotprod28/2, dotprod29/2, dotprod30/2
  dotprod1/1 -> Mux/1
  "IW{1,1}(2,:)'"/1 -> dotprod2/1
  dotprod2/1 -> Mux/2
  "IW{1,1}(3,:)'"/1 -> dotprod3/1
  dotprod3/1 -> Mux/3
  "IW{1,1}(4,:)'"/1 -> dotprod4/1
  dotprod4/1 -> Mux/4
  "IW{1,1}(5,:)'"/1 -> dotprod5/1
  dotprod5/1 -> Mux/5
  "IW{1,1}(6,:)'"/1 -> dotprod6/1
  dotprod6/1 -> Mux/6
  "IW{1,1}(7,:)'"/1 -> dotprod7/1
  dotprod7/1 -> Mux/7
  "IW{1,1}(8,:)'"/1 -> dotprod8/1
  dotprod8/1 -> Mux/8
  "IW{1,1}(9,:)'"/1 -> dotprod9/1
  dotprod9/1 -> Mux/9
  "IW{1,1}(10,:)'"/1 -> dotprod10/1
  dotprod10/1 -> Mux/10
  "IW{1,1}(11,:)'"/1 -> dotprod11/1
  dotprod11/1 -> Mux/11
  "IW{1,1}(12,:)'"/1 -> dotprod12/1
  dotprod12/1 -> Mux/12
  "IW{1,1}(13,:)'"/1 -> dotprod13/1
  dotprod13/1 -> Mux/13
  "IW{1,1}(14,:)'"/1 -> dotprod14/1
  dotprod14/1 -> Mux/14
  "IW{1,1}(15,:)'"/1 -> dotprod15/1
  dotprod15/1 -> Mux/15
  "IW{1,1}(16,:)'"/1 -> dotprod16/1
  dotprod16/1 -> Mux/16
  "IW{1,1}(17,:)'"/1 -> dotprod17/1
  dotprod17/1 -> Mux/17
  "IW{1,1}(18,:)'"/1 -> dotprod18/1
  dotprod18/1 -> Mux/18
  "IW{1,1}(19,:)'"/1 -> dotprod19/1
  dotprod19/1 -> Mux/19
  "IW{1,1}(20,:)'"/1 -> dotprod20/1
  dotprod20/1 -> Mux/20
  "IW{1,1}(21,:)'"/1 -> dotprod21/1
  dotprod21/1 -> Mux/21
  "IW{1,1}(22,:)'"/1 -> dotprod22/1
  dotprod22/1 -> Mux/22
  "IW{1,1}(23,:)'"/1 -> dotprod23/1
  dotprod23/1 -> Mux/23
  "IW{1,1}(24,:)'"/1 -> dotprod24/1
  dotprod24/1 -> Mux/24
  "IW{1,1}(25,:)'"/1 -> dotprod25/1
  dotprod25/1 -> Mux/25
  "IW{1,1}(26,:)'"/1 -> dotprod26/1
  dotprod26/1 -> Mux/26
  "IW{1,1}(27,:)'"/1 -> dotprod27/1
  dotprod27/1 -> Mux/27
  "IW{1,1}(28,:)'"/1 -> dotprod28/1
  dotprod28/1 -> Mux/28
  "IW{1,1}(29,:)'"/1 -> dotprod29/1
  dotprod29/1 -> Mux/29
  "IW{1,1}(30,:)'"/1 -> dotprod30/1
  dotprod30/1 -> Mux/30
  Mux/1 -> "iz{1,1}"/1

== system mrefrobotarm_previous_y_previous_u_previous_ref_cex_2/no_cex1/Layer 2/Delays 1 ==
  "p{2}" : Inport  PortDimensions=30
      mask Display: e = 0.06;c1 = [120 230 180]/255;c2 = ([120 230 180]+0)/(256+128);c3 = ([120 230 180]+128)/(256+128);patch([0 1 1 0],[0 0 1 1],c1);patch([0 1 1 1-e 1-e 0+e],[0 0 1 1-e 0+e 0+e],c2);patch([0 0 1 1-e 0+e 0+e],[0 1 1 1-e 1-e 0+e],c3);plot([0 1 1 0 0],[0 0 1 1 0]);
  mux : Mux  Inputs=1
      mask Display: e = 0.06;c1 = [120 150 230]/255;c2 = ([120 150 230]+0)/383;c3 = ([120 150 230]+128)/383;patch([0 1 1 0],[0 0 1 1],c1);patch([0 1 1 1-e 1-e 0+e],[0 0 1 1-e 0+e 0+e],c2);patch([0 0 1 1-e 0+e 0+e],[0 1 1 1-e 1-e 0+e],c3);plot([0 1 1 0 0],[0 0 1 1 0]);disp('Mux')
  "pd{2,1}" : Outport
      mask Display: e = 0.06;c1 = [120 230 180]/255;c2 = ([120 230 180]+0)/(256+128);c3 = ([120 230 180]+128)/(256+128);patch([0 1 1 0],[0 0 1 1],c1);patch([0 1 1 1-e 1-e 0+e],[0 0 1 1-e 0+e 0+e],c2);patch([0 0 1 1-e 0+e 0+e],[0 1 1 1-e 1-e 0+e],c3);plot([0 1 1 0 0],[0 0 1 1 0]);
  wires:
  "p{2}"/1 -> mux/1
  mux/1 -> "pd{2,1}"/1
